simulink subsystem "RX"  (R2022b)
settings: Solver=VariableStepAuto  StartTime=0.0  StopTime=10.0  RelTol=1e-3
settings Model: Creator=Ali-Laptop  LastModifiedBy=Ali-Laptop

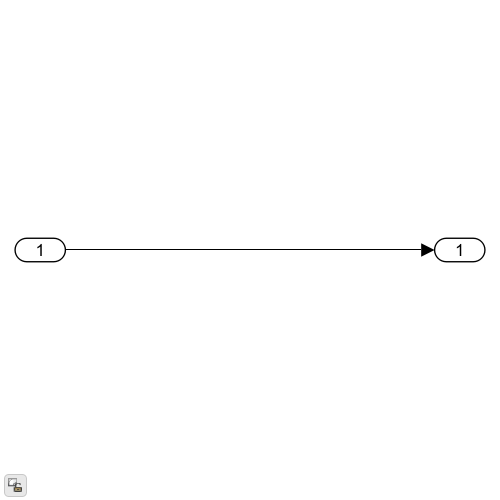
[thumbnail: Simulink's stored preview of the top-level diagram]
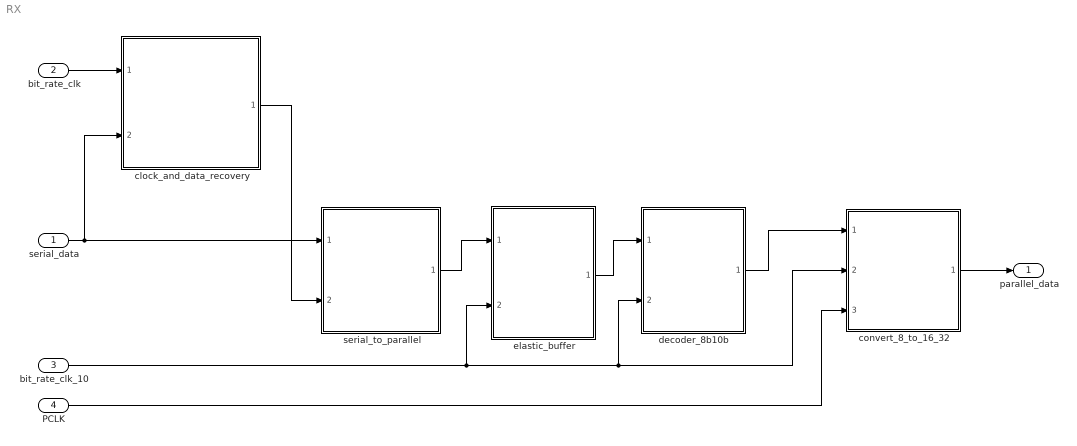
== system RX ==
  serial_data : Inport
  bit_rate_clk : Inport  Port=2
  bit_rate_clk_10 : Inport  Port=3
  PCLK : Inport  Port=4
  clock_and_data_recovery : Subsystem  ReferencedSubsystem=clock_and_data_recovery
  convert_8_to_16_32 : Subsystem  ReferencedSubsystem=convert_8_to_16_32
  decoder_8b10b : Subsystem  ReferencedSubsystem=decoder_8b10b
  elastic_buffer : Subsystem  ReferencedSubsystem=elastic_buffer
  serial_to_parallel : Subsystem  ReferencedSubsystem=serial_to_parallel
  parallel_data : Outport
  wires:
  serial_to_parallel/1 -> elastic_buffer/1
  elastic_buffer/1 -> decoder_8b10b/1
  convert_8_to_16_32/1 -> parallel_data/1
  clock_and_data_recovery/1 -> serial_to_parallel/2
  bit_rate_clk/1 -> clock_and_data_recovery/1
  serial_data/1 -> clock_and_data_recovery/2, serial_to_parallel/1
  bit_rate_clk_10/1 -> elastic_buffer/2, decoder_8b10b/2, convert_8_to_16_32/2
  PCLK/1 -> convert_8_to_16_32/3
  decoder_8b10b/1 -> convert_8_to_16_32/1
